simulink model "Examples_Session_1"  (R2023b)
settings: Solver=VariableStepAuto  StartTime=0.0  StopTime=10.0  RelTol=1e-3
libraries: simulink x1
settings Model: Creator=hp  LastModifiedBy=hp

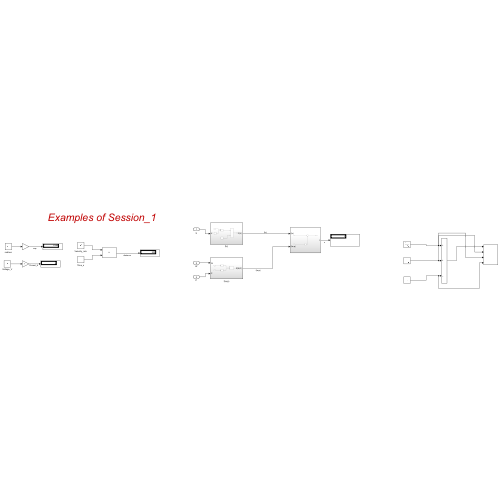
[thumbnail: Simulink's stored preview of the top-level diagram]
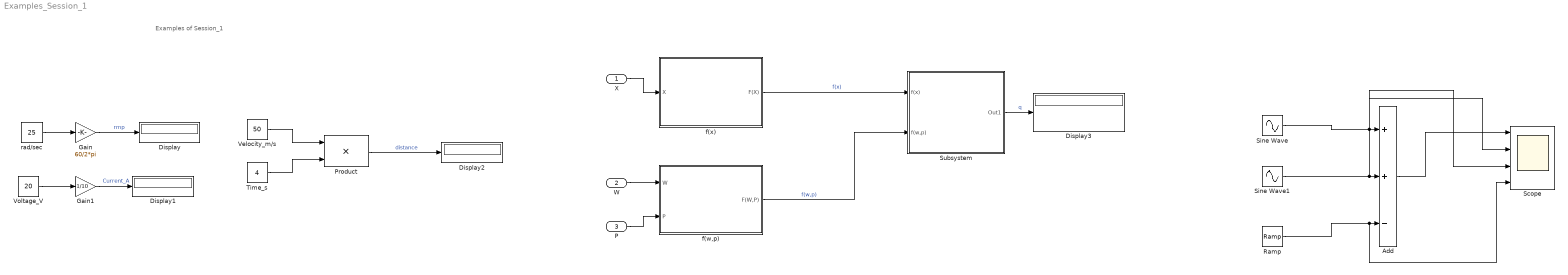
== system Examples_Session_1 ==
  note: Examples of Session_1
  X : Inport
  W : Inport  Port=2
  P : Inport  Port=3
  Add : Sum  Inputs=++-
  Display{,1..3} (4 alike) : Display
  Gain : Gain  Gain=60/2*pi
  Gain1 : Gain  Gain=1/10
  Product : Product
  Ramp : simulink/Sources/Ramp  slope=1  start=0  InitialOutput=0
  Scope : Scope  NumInputPorts=4
  Sine Wave : Sin  Frequency=5  SampleTime=0
  Sine Wave1 : Sin  Frequency=3  SampleTime=0
  Subsystem : Subsystem
  Time_s : Constant  Value=4
  Velocity_m/s : Constant  Value=50
  Voltage_V : Constant  Value=20
  f(w,p) : Subsystem
  f(x) : Subsystem
  rad/sec : Constant  Value=25
  wires:
  rad/sec/1 -> Gain/1
  Gain/1 -> Display/1  "rmp"
  Gain1/1 -> Display1/1  "Current_A"
  Voltage_V/1 -> Gain1/1
  Velocity_m/s/1 -> Product/1
  Time_s/1 -> Product/2
  Product/1 -> Display2/1  "distance"
  X/1 -> f(x)/1(X)
  W/1 -> f(w,p)/1(W)
  P/1 -> f(w,p)/2(P)
  f(x)/1(F(X)) -> Subsystem/1(f(x))  "f(x)"
  f(w,p)/1(F(W,P)) -> Subsystem/2(f(w,p))  "f(w,p)"
  Subsystem/1(Out1) -> Display3/1  "q"
  Sine Wave/1 -> Scope/2, Add/1
  Sine Wave1/1 -> Scope/3, Add/2
  Ramp/1 -> Scope/4, Add/3
  Add/1 -> Scope/1

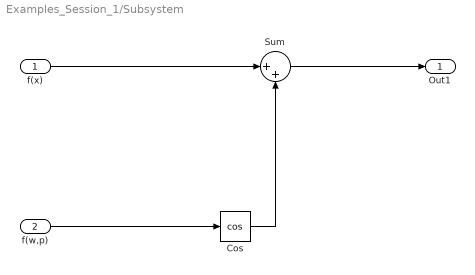
== system Examples_Session_1/Subsystem ==
  f(x) : Inport
  f(w,p) : Inport  Port=2
  Cos : Trigonometry  Operator=cos
  Sum : Sum  Inputs=|++
  Out1 : Outport
  wires:
  f(x)/1 -> Sum/1
  Cos/1 -> Sum/2
  f(w,p)/1 -> Cos/1
  Sum/1 -> Out1/1

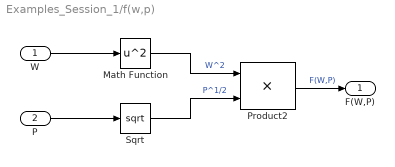
== system Examples_Session_1/f(w,p) ==
  W : Inport
  P : Inport  Port=2
  Math Function : Math  Operator=square
  Product2 : Product
  Sqrt : Sqrt
  F(W,P) : Outport
  wires:
  Math Function/1 -> Product2/1  "W^2"
  P/1 -> Sqrt/1
  Product2/1 -> F(W,P)/1  "F(W,P)"
  Sqrt/1 -> Product2/2  "P^1/2"
  W/1 -> Math Function/1

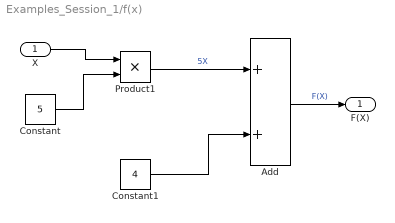
== system Examples_Session_1/f(x) ==
  X : Inport
  Add : Sum
  Constant : Constant  Value=5
  Constant1 : Constant  Value=4
  Product1 : Product
  F(X) : Outport
  wires:
  Constant/1 -> Product1/2
  Product1/1 -> Add/1  "5X"
  X/1 -> Product1/1
  Add/1 -> F(X)/1  "F(X)"
  Constant1/1 -> Add/2
